simulink model "P1_pt1"  (R2023b)
settings: Solver=ode4  StartTime=0.0  StopTime=25  FixedStep=0.1  RelTol=1e-3
undefined symbols (not defined in the file): A, b, J, w_0
settings Model: Creator=oscar  LastModifiedBy=oscar

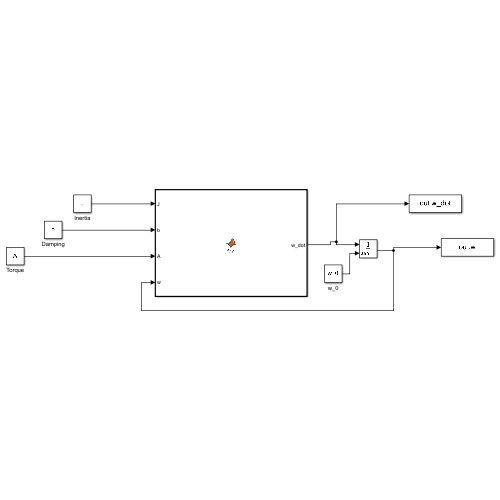
[thumbnail: Simulink's stored preview of the top-level diagram]
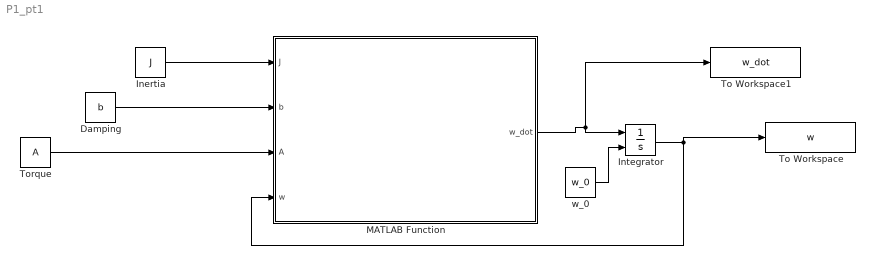
== system P1_pt1 ==
  Damping : Constant  Value=b
  Inertia : Constant  Value=J
  Integrator : Integrator  InitialConditionSource=external
  MATLAB Function : MATLAB Function  TreatAsAtomicUnit=on
  To Workspace : ToWorkspace  VariableName=w  SaveFormat=Timeseries  SampleTime=-1
  To Workspace1 : ToWorkspace  VariableName=w_dot  SaveFormat=Timeseries  SampleTime=-1
  Torque : Constant  Value=A
  w_0 : Constant  Value=w_0
  wires:
  MATLAB Function/1(w_dot) -> To Workspace1/1, Integrator/1
  Inertia/1 -> MATLAB Function/1(J)
  Damping/1 -> MATLAB Function/2(b)
  Torque/1 -> MATLAB Function/3(A)
  Integrator/1 -> To Workspace/1, MATLAB Function/4(w)
  w_0/1 -> Integrator/2

== matlab function P1_pt1/MATLAB Function ==
  data: J input; w_dot output; b input; A input; w input
function w_dot = fcn(J, b, A, w)

w_dot = (1/J)*(A-(b*w));

end
